simulink model "lr_disc_all"  (R2015a)
settings: Solver=ode45  StartTime=0.0  StopTime=.04  MaxStep=Ts/1000  RelTol=1e-3
values from neighbouring files (symbols this model uses):
  alphac = 2*pi*300    (= 1884.95559215)    [Sim_lr_disc_all.m]
  iData = (c0 + cS*abs(psiData).^S).*psiData    [Sim_lr_disc_all.m]
  invLData = c0 + cS*abs(psiData).^S    [Sim_lr_disc_all.m]
  R = RAct    (= 3)    [Sim_lr_disc_all.m]
  sigmaNoise = 0*.01    (= 0)    [Sim_lr_disc_all.m]
  TNoise = Ts    (= 0.0004)    [Sim_lr_disc_all.m]
  Ts = 400e-6    (= 0.0004)    [Sim_lr_disc_all.m]
  Tsw = Ts    (= 0.0004)    [Sim_lr_disc_all.m]
  Udc = 350    [Sim_lr_disc_all.m]
  uMax = Udc    (= 350)    [Sim_lr_disc_all.m]
undefined symbols (not defined in the file): c0Act, cSAct, RAct, SAct
libraries: simulink x2
settings Model: Creator=mhink  LastModifiedBy=mhinkkan
settings DataIOCC: SaveFormat=Dataset
settings HardwareCC: ProdBitPerPointer=64  ProdLargestAtomicFloat=Float  ProdIntDivRoundTo=Zero  ProdEndianess=LittleEndian  ProdHWDeviceType=Specified
settings GRTTargetCC: GeneratePreprocessorConditionals=Use local settings

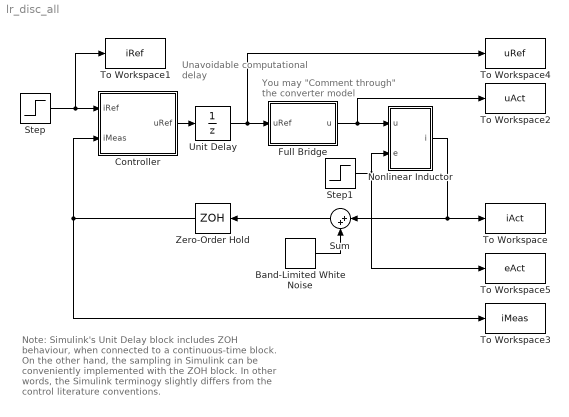
== system lr_disc_all ==
  note: Unavoidable
      | computational
      | delay
  note: Note:
      |
      | Simulink's Unit Delay block includes ZOH behaviour,
      | when connected to a continuous-time block.
      |
      | On the other hand, the sampling in Simulink can be
      | conveniently implemented with the ZOH block.
      |
      | In other words, the Simulink terminogy slightly
      | differs from the control literature conventions.
  note: You may "Comment through"
      | the converter model
  Band-Limited White Noise : simulink/Sources/Band-Limited White Noise  Cov=[sigmaNoise^2*TNoise]  Ts=TNoise  seed=[23341]
  Controller : Subsystem
  Full Bridge : Subsystem
  Nonlinear Inductor : Subsystem  mask{R=RAct, c0=c0Act, cS=cSAct, S=SAct}
      mask prompts: R "Resistance R (ohm)"; c0 "Inverse of the unsaturated inductance c0 (1/H)"; cS "Saturation model parameter cS (1/(Vs)^S)"; S "Saturation model exponent S"
  Step : Step  Time=2e-3  After=10  SampleTime=Ts
  Step1 : Step  Time=20e-3  After=100  SampleTime=0
  Sum : Sum  Inputs=|++
  To Workspace : ToWorkspace  VariableName=iAct  SaveFormat=Timeseries  SampleTime=-1
  To Workspace1 : ToWorkspace  VariableName=iRef  SaveFormat=Timeseries  SampleTime=-1
  To Workspace2 : ToWorkspace  VariableName=uAct  SaveFormat=Timeseries  SampleTime=-1
  To Workspace3 : ToWorkspace  VariableName=iMeas  SaveFormat=Timeseries  SampleTime=-1
  To Workspace4 : ToWorkspace  VariableName=uRef  SaveFormat=Timeseries  SampleTime=-1
  To Workspace5 : ToWorkspace  VariableName=eAct  SaveFormat=Timeseries  SampleTime=-1
  Unit Delay : UnitDelay  SampleTime=Ts
  Zero-Order Hold : ZeroOrderHold  SampleTime=Ts
  wires:
  Step/1 -> Controller/1(iRef), To Workspace1/1
  Step1/1 -> Nonlinear Inductor/2(e), To Workspace5/1
  Zero-Order Hold/1 -> Controller/2(iMeas), To Workspace3/1
  Controller/1(uRef) -> Unit Delay/1
  Unit Delay/1 -> Full Bridge/1(uRef), To Workspace4/1
  Full Bridge/1(u) -> Nonlinear Inductor/1(u), To Workspace2/1
  Nonlinear Inductor/1(i) -> To Workspace/1, Sum/1
  Sum/1 -> Zero-Order Hold/1
  Band-Limited White Noise/1 -> Sum/2

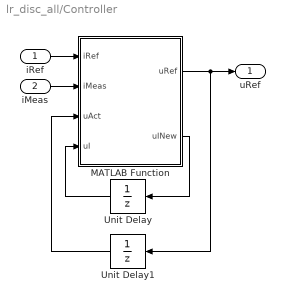
== system lr_disc_all/Controller ==
  iRef : Inport
  iMeas : Inport  Port=2
  MATLAB Function : MATLAB Function  TreatAsAtomicUnit=on
      settings: PermitHierarchicalResolution=ParametersOnly
  Unit Delay : UnitDelay  SampleTime=Ts
  Unit Delay1 : UnitDelay  SampleTime=Ts
  uRef : Outport
  wires:
  MATLAB Function/2(uINew) -> Unit Delay/1
  Unit Delay/1 -> MATLAB Function/4(uI)
  iRef/1 -> MATLAB Function/1(iRef)
  iMeas/1 -> MATLAB Function/2(iMeas)
  Unit Delay1/1 -> MATLAB Function/3(uAct)
  MATLAB Function/1(uRef) -> uRef/1, Unit Delay1/1

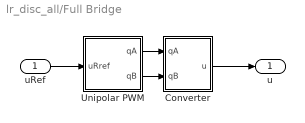
== system lr_disc_all/Full Bridge ==
  uRef : Inport
  Converter : Subsystem
  Unipolar PWM : Subsystem
  u : Outport
  wires:
  Converter/1(u) -> u/1
  Unipolar PWM/2(qB) -> Converter/2(qB)
  Unipolar PWM/1(qA) -> Converter/1(qA)
  uRef/1 -> Unipolar PWM/1(uRref)

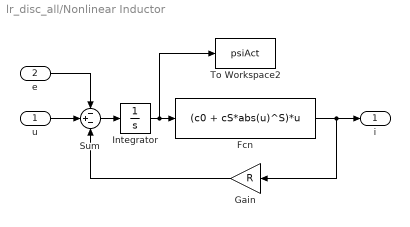
== system lr_disc_all/Nonlinear Inductor ==
  u : Inport
  e : Inport  Port=2
  Fcn : Fcn  Expr=(c0 + cS*abs(u)^S)*u
  Gain : Gain  Gain=R
  Integrator : Integrator
  Sum : Sum  Inputs=-+-
  To Workspace2 : ToWorkspace  VariableName=psiAct  SaveFormat=Timeseries  SampleTime=-1
  i : Outport
  wires:
  u/1 -> Sum/2
  Integrator/1 -> To Workspace2/1, Fcn/1
  Sum/1 -> Integrator/1
  Fcn/1 -> i/1, Gain/1
  e/1 -> Sum/1
  Gain/1 -> Sum/3

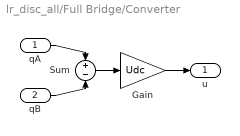
== system lr_disc_all/Full Bridge/Converter ==
  qA : Inport
  qB : Inport  Port=2
  Gain : Gain  Gain=Udc
  Sum : Sum  Inputs=+|-
  u : Outport
  wires:
  qA/1 -> Sum/1
  qB/1 -> Sum/2
  Gain/1 -> u/1
  Sum/1 -> Gain/1

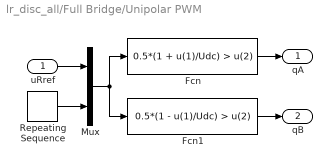
== system lr_disc_all/Full Bridge/Unipolar PWM ==
  uRref : Inport
  Fcn : Fcn  Expr=0.5*(1 + u(1)/Udc) > u(2)
  Fcn1 : Fcn  Expr=0.5*(1 - u(1)/Udc) > u(2)
  Mux : Mux  Inputs=2
  Repeating Sequence : simulink/Sources/Repeating Sequence  rep_seq_t=Tsw*[0 0.5 1]  rep_seq_y=[1 0 1]
  qA : Outport
  qB : Outport  Port=2
  wires:
  uRref/1 -> Mux/1
  Mux/1 -> Fcn1/1, Fcn/1
  Repeating Sequence/1 -> Mux/2
  Fcn/1 -> qA/1
  Fcn1/1 -> qB/1

== matlab function lr_disc_all/Controller/MATLAB Function ==
  data: iRef input; uRef output; iMeas input; uAct input; uI input; uINew output; uMax parameter; alphac parameter; Ts parameter; iData parameter; invLData parameter; R parameter
function [uRef,uINew] = fcn(iRef,iMeas,uAct,uI,uMax,alphac,Ts, iData, invLData, R)

MODE = 5;

% Fetch inverse inductances from a look-up table 
% Inverse inductance is convenient for interpolation and extrapolation
invLMeas = interp1(iData,invLData,abs(iMeas),'linear','extrap');
invLRef = interp1(iData,invLData,abs(iRef),'linear','extrap');

switch MODE
    case 1
        % Type: PI controller 
        % Design: continuous
        % State variable: current 

       % Controller gains        
        kt = alphac/invLMeas; k1 = kt; ki = Ts*alphac*R; k2 = 0; 
        
    case 2
        % Type: state feedback 
        % Design: continuous
        % State variable: current 

       % Controller gains        
        kt = alphac/invLMeas; k1 = 2*alphac/invLMeas - R; 
        ki = Ts*alphac^2/invLMeas; k2 = 0; 

    case 3
        % Type: state feedback 
        % Design: direct discrete
        % State variable: current 
        ad = exp(-R*invLMeas*Ts); bd = (1 - ad)/(R*invLMeas);
        
        % Controller gains        
        beta = exp(-alphac*Ts);
        a0 = 0; a1 = beta^2; a2 = -2*beta; b1 = 1 - beta;
        kt = b1/(invLMeas*bd); k2 = a2 + ad + 1; 
        k1 = (a1 - ad*(1 - k2) + k2)/(invLMeas*bd); 
        ki = k1 + (a0 - k2*ad)/(invLMeas*bd);

    case 4
        % Type: state feedback 
        % Design: continuous
        % State variable: flux linkage 
        
        % Change the state variable
        psiMeas = iMeas/invLMeas; psiRef = iRef/invLRef; 
    
        % Controller gains        
        kt = alphac; k1 = 2*alphac - R*invLMeas; 
        ki = Ts*alphac^2; k2 = 0; 

    case 5
        % Type: state feedback 
        % Design: direct discrete
        % State variable: flux linkage 

        % Change the state variable
        psiMeas = iMeas/invLMeas; psiRef = iRef/invLRef; 

        % Discrete-time model
        ad = exp(-R*invLMeas*Ts); invbd = R*invLMeas/(1 - ad);
        
        % Controller gains
        beta = exp(-alphac*Ts);
        a0 = 0; a1 = beta^2; a2 = -2*beta; b1 = 1 - beta;
        k2 = a2 + ad + 1; 
        k1 = (a1 - ad*(1 - k2) + k2)*invbd; 
        ki = k1 + (a0 - k2*ad)*invbd;
        kt = b1*invbd; 
end

% Calculate the ideal controller output
switch MODE
    case {1, 2, 3}
        % State variable: current
        uRefIdeal = kt*iRef - k1*iMeas - k2*uAct + uI;
    otherwise
        % State variable: flux linkage
        uRefIdeal = kt*psiRef - k1*psiMeas - k2*uAct + uI;        
end

% Limit the output
uRef = uRefIdeal;
if(uRef > uMax)
    uRef = uMax;
elseif(uRef < -uMax)
    uRef = -uMax;
end

% Update the integrator state. Last term is the antiwindup.
switch MODE
    case {1, 2, 3}
        % State variable: current
        uINew = uI + ki*((iRef - iMeas) + (uRef - uRefIdeal)/kt);
    otherwise
        % State variable: flux linkage
        uINew = uI + ki*((psiRef - psiMeas) + (uRef - uRefIdeal)/kt);
end
